simulink model "Ex1_gravidade"  (R2015a)
settings: Solver=ode45  StartTime=0.0  StopTime=10.0  RelTol=1e-3
values from neighbouring files (symbols this model uses):
  A = [0 1 0 0; -k1/M1 -d/M1 k1/M1 d/M1; 0 0 0 1; k1/M2 d/M2 -(k1+k2)/M2 -d/M2]    [ex1.m]
  B = [0 0 0 k2/M2; 0 g 0 g]'    [ex1.m]
  C = [1 0 0 0 ; 0 0 1 0]    [ex1.m]
  D = [0 0 ; 0 0 ]    [ex1.m]
settings Model: Creator=martinspedro  LastModifiedBy=martinspedro

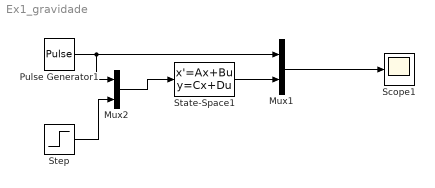
== system Ex1_gravidade ==
  Mux1 : Mux  Inputs=2
  Mux2 : Mux  Inputs=2
  Pulse Generator1 : DiscretePulseGenerator  PulseType=Time based  Amplitude=0.2  Period=0.3  PulseWidth=50
  Scope1 : Scope
      settings: ShowLegends=on
  State-Space1 : StateSpace  A=A  B=B  C=C  D=D  X0=0
  Step : Step  Time=0  SampleTime=0
  wires:
  Mux1/1 -> Scope1/1
  State-Space1/1 -> Mux1/2
  Pulse Generator1/1 -> Mux2/1, Mux1/1
  Mux2/1 -> State-Space1/1
  Step/1 -> Mux2/2
